simulink model "sedemo_tank_filling_station"  (Simulink 7.5)
settings: Solver=ode45  StartTime=0.0  StopTime=500  MaxStep=inf  RelTol=1e-3
undefined symbols (not defined in the file or in its folder): des_subsystemblock, des_subsysteminport, des_subsystemoutport, des_subsystemsupportblock
libraries: simeventsgenerators1 x3, simeventsattributes2 x2, simeventstranslate1 x2, simeventssignalmanage1 x2, simeventssink1 x1, simeventsinfo x1, simeventsserver1 x1, simeventsqueue1 x1
settings Model: Creator=The MathWorks Inc.  ExtModeAutoUpdateStatusClock=off
settings SolverCC: ZeroCrossControl=EnableAll
settings DataIOCC: SaveOutput=off  SaveTime=off
settings OptimizationCC: InlineInvariantSignals=on  InitFltsAndDblsToZero=on  EfficientMapNaN2IntZero=off
settings DebuggingCC: AlgebraicLoopMsg=error  SaveWithParameterizedLinksMsg=none  SignalResolutionControl=TryResolveAllWithWarning  SolverPrmCheckMsg=none  MultiTaskDSMMsg=warning  MultiTaskCondExecSysMsg=none  SigSpecEnsureSampleTimeMsg=none  InvalidFcnCallConnMsg=warning  BusObjectLabelMismatch=none  StrictBusMsg=None
settings RTWCC: IncludeERTFirstTime=on
settings GRTTargetCC: TargetFcnLib=ansi_tfl_tmw.mat
settings SimEventsCC: propIdentEventSeed=12345678  propDiagAttribOutput=1  propDiagFcnCallOutput=1  propDiagStatOutput=0

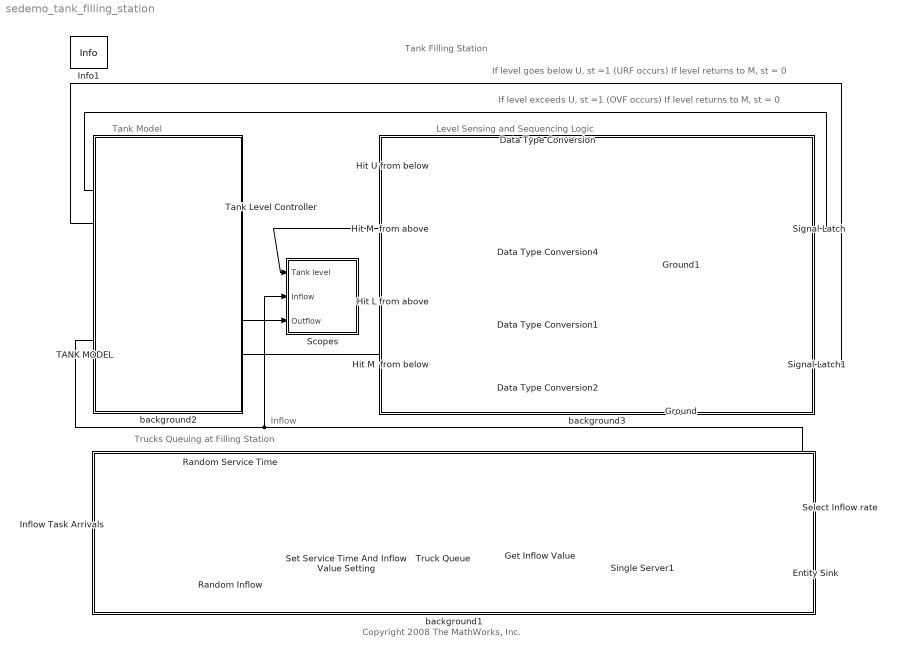
== system sedemo_tank_filling_station ==
  note: If level exceeds U, st =1 (OVF occurs)
      | If level returns to M, st = 0
  note: If level goes below U, st =1 (URF occurs)
      | If level returns to M, st = 0
  note: Tank Filling Station
  note: Trucks Queuing at Filling Station
  note: Tank Model
  note: Level Sensing and Sequencing Logic
  note: Inflow
  note: Copyright 2008 The MathWorks, Inc.
  Data Type Conversion{,1..2,4} (4 alike) : DataTypeConversion  OutDataType=sfix(16)  OutScaling=2^0
  Entity Sink : simeventssink1/Entity Sink  Priority=1  SystemSampleTime=-1  AvailableForArrivals=on  StatNumberArrived=Off
  Get Inflow Value : simeventsattributes2/Get Attribute  Priority=1  DialogController=des_ddg_create  DialogControllerArgs=DataTag2  SystemSampleTime=-1  AttributeName=Inflow  AttributeMissing=Error  AttributeDefaultValue=0  AttributeSendTiming=After entity departure  AttributeTreatAsVector=1  StatNumberDeparted=Off  EvaluatedDefaultAttributeValue={[]}
  Ground : Ground
  Ground1 : Ground
  Hit L from above : HitCross  HitCrossingOffset=1  HitCrossingDirection=falling
  Hit M  from above : HitCross  HitCrossingOffset=3  HitCrossingDirection=falling
  Hit M  from below : HitCross  HitCrossingOffset=3  HitCrossingDirection=rising
  Hit U from below : HitCross  HitCrossingOffset=5  HitCrossingDirection=rising
  Inflow Task Arrivals : simeventsgenerators1/Entity Generators/Time-Based Entity Generator  Priority=1  DialogController=des_ddg_create  DialogControllerArgs=DataTag4  SystemSampleTime=-1  GenerateEntitiesUpon=Intergeneration time from dialog  Distribution=Exponential  Minimum=0  Maximum=8  Mean=1.2  InitialSeed=375501  Period=12  PriorityEntityGeneration=301  GenerateEntityAtSimulationStart=on  ResponseWhenBlocked=Pause generation  ResponseWhenUnblocked=Immediate restart  EntityType=Standard  StatNumberDeparted=Off  StatPendingEntity=Off  StatAverageIntergenerationTime=Off
  Info1 : simeventsinfo/Info  SystemSampleTime=-1
  Random Inflow : simeventsgenerators1/Signal Generators/Event-Based Random Number  SystemSampleTime=-1  distribution=Uniform  meanExp=1  minUnif=10  maxUnif=20  pOneBern=0.25  pSuccessBino=0.5  numTrialBino=1  meanNorm=0  stdNorm=1  minTri=1  maxTri=3  modeTri=2  thresholdLogn=0  scaleLogn=1  shapeLogn=1  pSuccessGeo=0.5  meanPoiss=1  thresholdLogl=0  scaleLogl=1  thresholdGam=0  scaleGam=1  shapeGam=1  minBeta=0  maxBeta=1  shape1Beta=1  shape2Beta=1  minUnid=1  maxUnid=20  numValueUnid=20  thresholdWbl=0  scaleWbl=1  shapeWbl=1  valueVecCont=[0 1]  cdfVecCont=[0 1]  valueVecDisc=[1 2]  probVecDisc=[0.2 0.8]  seed=8023  IsProcessed=on  isConnected=1
  Random Service Time : simeventsgenerators1/Signal Generators/Event-Based Random Number  SystemSampleTime=-1  distribution=Beta  meanExp=1  minUnif=10  maxUnif=20  pOneBern=0.25  pSuccessBino=0.5  numTrialBino=1  meanNorm=0  stdNorm=1  minTri=1  maxTri=3  modeTri=2  thresholdLogn=0  scaleLogn=1  shapeLogn=1  pSuccessGeo=0.5  meanPoiss=1  thresholdLogl=0  scaleLogl=1  thresholdGam=0  scaleGam=1  shapeGam=1  minBeta=.75  maxBeta=1.25  shape1Beta=1  shape2Beta=1  minUnid=1  maxUnid=20  numValueUnid=20  thresholdWbl=0  scaleWbl=1  shapeWbl=1  valueVecCont=[0 1]  cdfVecCont=[0 1]  valueVecDisc=[1 2]  probVecDisc=[0.2 0.8]  seed=9231  IsProcessed=on  isConnected=1
  Scopes : Subsystem
      settings: RequestExecContextInheritance=on
  Select Inflow rate : Subsystem  LoadFcn=des_subsystemblock(gcb, 'load');  InitFcn=des_subsystemblock(gcb, 'init');  StartFcn=des_subsystemblock(gcb, 'start');  StopFcn=des_subsystemblock(gcb, 'stop');
      settings: CopyFcn=des_subsystemblock(gcb, 'copy');  DeleteFcn=des_subsystemblock(gcb, 'delete');  UndoDeleteFcn=des_subsystemblock(gcb, 'undodelete');  ModelCloseFcn=des_subsystemblock(gcb, 'modelclose');  PreSaveFcn=des_subsystemblock(gcb, 'presave');  NameChangeFcn=des_subsystemblock(gcb, 'namechange');  ParentCloseFcn=des_subsystemblock(gcb, 'parentclose');  ErrorFcn=des_subsystemerror
  Set Service Time And Inflow Value Setting : simeventsattributes2/Set Attribute  Priority=1  DialogController=des_ddg_create  DialogControllerArgs=DataTag15  SystemSampleTime=-1  AttributeFrom=Signal port|Signal port  AttributeName=ServiceTime|Inflow  AttributeTreatAsVector=1|1  AttributeValue=1|0  AttributeCreate=on  StatNumberDeparted=Off  EvaluatedAttributeValue={[];[]}
  Signal Latch : simeventssignalmanage1/Signal Latch  Priority=1  SystemSampleTime=-1  InitialMemoryValue=0  WriteMemoryUpon=Change in signal from port wvc  MemoryWriteEdgeOption=Rising  SpecifyWriteEventPriority=on  PriorityMemoryWrite=7100  ReadMemoryUpon=Change in signal from port rvc  MemoryReadEdgeOption=Falling  SpecifyReadEventPriority=on  PriorityMemoryRead=7000  ReportMemoryState=on  ReportMemoryUponWrite=off  ReportMemoryUponRead=off
  Signal Latch1 : simeventssignalmanage1/Signal Latch  Priority=1  SystemSampleTime=-1  InitialMemoryValue=0  WriteMemoryUpon=Change in signal from port wvc  MemoryWriteEdgeOption=Rising  SpecifyWriteEventPriority=on  PriorityMemoryWrite=7100  ReadMemoryUpon=Change in signal from port rvc  MemoryReadEdgeOption=Falling  SpecifyReadEventPriority=on  PriorityMemoryRead=7000  ReportMemoryState=on  ReportMemoryUponWrite=off  ReportMemoryUponRead=off
  Single Server1 : simeventsserver1/Single Server  Priority=1  SystemSampleTime=-1  ServiceTimeFrom=Attribute  ServiceTime=2  AttributeName=ServiceTime  PriorityServiceCompletion=500  PermitPreemption=off  SortingAttributeName=PriorityAttributeName  SortingDirection=Ascending  WriteToAttribute=off  ResidualAttributeName=ResidualServiceTime  CreateAttribute=on  EnableTOPort=off  StatNumberDeparted=Off  StatNumberInBlock=On  StatNumberPreempted=Off  StatPendingEntity=Off  StatAverageWait=Off  StatUtilization=Off  StatNumberTimedout=Off
  TANK MODEL : Subsystem
  Tank Level Controller : Subsystem
  Truck Queue : simeventsqueue1/FIFO Queue  Priority=1  SystemSampleTime=-1  Capacity=2500  EnableTOPort=off  StatNumberDeparted=Off  StatNumberInBlock=Off  StatPendingEntity=Off  StatAverageWait=Off  StatAverageQueueLength=Off  StatNumberTimedout=Off
  background1 : Subsystem
      mask Display: disp('')
  background2 : Subsystem
      mask Display: disp('')
  background3 : Subsystem
      mask Display: disp('')
  wires:
  Signal Latch/1 -> Tank Level Controller/1(OVF state)
  Signal Latch1/1 -> Tank Level Controller/2(URF state)
  Select Inflow rate/1(Inflow) -> TANK MODEL/1(Inflow), Scopes/2(Inflow)
  Hit U from below/1 -> Data Type Conversion/1
  Hit L from above/1 -> Data Type Conversion1/1
  Hit M  from above/1 -> Data Type Conversion4/1
  Tank Level Controller/1(Outflow) -> TANK MODEL/2(Outflow), Scopes/3(Outflow)
  Hit M  from below/1 -> Data Type Conversion2/1
  Ground/1 -> Signal Latch1/3
  Random Inflow/1 -> Set Service Time And Inflow Value Setting/2
  Get Inflow Value/1 -> Select Inflow rate/1(Inflow Value)
  Single Server1/1 -> Select Inflow rate/2(Server State)
  Random Service Time/1 -> Set Service Time And Inflow Value Setting/1
  Data Type Conversion/1 -> Signal Latch/1
  Data Type Conversion4/1 -> Signal Latch/2
  Ground1/1 -> Signal Latch/3
  Data Type Conversion1/1 -> Signal Latch1/1
  Data Type Conversion2/1 -> Signal Latch1/2
  TANK MODEL/1(Tank Level) -> Hit M  from below/1, Hit L from above/1, Hit M  from above/1, Hit U from below/1, Scopes/1(Tank level)
  connections:
  Entity Sink/LConn1 -- Single Server1/RConn1
  Set Service Time And Inflow Value Setting/RConn1 -- Truck Queue/LConn1
  Truck Queue/RConn1 -- Get Inflow Value/LConn1
  Get Inflow Value/RConn1 -- Single Server1/LConn1
  Inflow Task Arrivals/RConn1 -- Set Service Time And Inflow Value Setting/LConn1

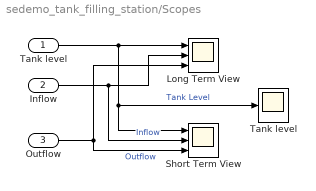
== system sedemo_tank_filling_station/Scopes ==
  Tank level : Inport  OutDataType=sfix(16)  OutScaling=2^0
  Inflow : Inport  Port=2  OutDataType=sfix(16)  OutScaling=2^0
  Outflow : Inport  Port=3  OutDataType=sfix(16)  OutScaling=2^0
  Long Term View : Scope  NumInputPorts=3
      settings: DeleteFcn=simscope BlockIsBeingDestroyed  TickLabels=on  TimeRange=500  YMin=0.5~0~10  YMax=5.5~20~20
  Short Term View : Scope  NumInputPorts=3
      settings: DeleteFcn=simscope BlockIsBeingDestroyed  TickLabels=on  TimeRange=50  YMin=0.5~0~10  YMax=5.5~20~20
  "Tank level " : Scope
      settings: DeleteFcn=simscope BlockIsBeingDestroyed  TickLabels=on  TimeRange=500  YMin=0.5  YMax=5.5  SaveName=ScopeData2
  wires:
  Tank level/1 -> Long Term View/1, Short Term View/1, "Tank level "/1  "Tank Level"
  Inflow/1 -> Long Term View/2, Short Term View/2  "Inflow"
  Outflow/1 -> Short Term View/3, Long Term View/3  "Outflow"

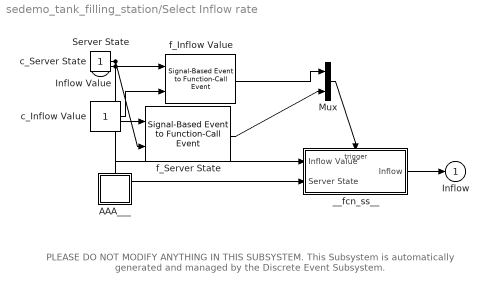
== system sedemo_tank_filling_station/Select Inflow rate ==
  note: PLEASE DO NOT MODIFY ANYTHING IN THIS SUBSYSTEM.
      | This Subsystem is automatically generated and
      | managed by the Discrete Event Subsystem.
  Inflow Value : Inport  DataType=double  OutDataType=sfix(16)  OutScaling=2^0  OutDataTypeStr=double
  Server State : Inport  Port=2  DataType=double  OutDataType=sfix(16)  OutScaling=2^0  OutDataTypeStr=double
  AAA___ : Subsystem  LoadFcn=des_subsystemsupportblock(gcb, 'load');  InitFcn=des_subsystemsupportblock(gcb, 'init');  StartFcn=des_subsystemsupportblock(gcb, 'start');  StopFcn=des_subsystemsupportblock(gcb, 'stop');
      settings: CopyFcn=des_subsystemsupportblock(gcb, 'copy');  DeleteFcn=des_subsystemsupportblock(gcb, 'delete');  UndoDeleteFcn=des_subsystemsupportblock(gcb, 'undodelete');  ModelCloseFcn=des_subsystemsupportblock(gcb, 'modelclose');  PreSaveFcn=des_subsystemsupportblock(gcb, 'presave');  NameChangeFcn=des_subsystemsupportblock(gcb, 'namechange');  OpenFcn=des_subsystemsupportblock(gcb, 'open');  ParentCloseFcn=des_subsystemsupportblock(gcb, 'parentclose');
  Mux : Mux  Inputs=2
  __fcn_ss__ : Subsystem  TreatAsAtomicUnit=on
      settings: PropExecContextOutsideSubsystem=on
  c_Inflow Value : Constant  OutDataType=sfix(16)  OutScaling=2^0
  c_Server State : Constant  OutDataType=sfix(16)  OutScaling=2^0
  f_Inflow Value : simeventstranslate1/Signal-Based Event to Function-Call Event  Priority=1  SystemSampleTime=-1  GenerateFunctionCallUpon=Sample time hit from port ts  SignalEdgeOption=Rising  EnableE1Port=on  EnableF2Port=off  EnableE2Port=off  SpecifyEventPriority=off  PriorityFunctionCall=20  FunctionCallDelayFrom=Dialog  DelayFunctionCall=0  StatNumberF1Calls=Off  StatNumberF2Calls=Off  MaskBlockType=DESS_EVENT_PORT
  f_Server State : simeventstranslate1/Signal-Based Event to Function-Call Event  Priority=1  SystemSampleTime=-1  GenerateFunctionCallUpon=Sample time hit from port ts  SignalEdgeOption=Rising  EnableE1Port=on  EnableF2Port=off  EnableE2Port=off  SpecifyEventPriority=off  PriorityFunctionCall=20  FunctionCallDelayFrom=Dialog  DelayFunctionCall=0  StatNumberF1Calls=Off  StatNumberF2Calls=Off  MaskBlockType=DESS_EVENT_PORT
  Inflow : Outport  OutDataType=sfix(16)  OutScaling=2^0
  wires:
  __fcn_ss__/1(Inflow) -> Inflow/1
  f_Inflow Value/1 -> Mux/1
  c_Inflow Value/1 -> f_Inflow Value/2
  Mux/1 -> __fcn_ss__/Trigger
  f_Server State/1 -> Mux/2
  c_Server State/1 -> f_Server State/2
  Inflow Value/1 -> f_Inflow Value/1, __fcn_ss__/1(Inflow Value)
  Server State/1 -> f_Server State/1, __fcn_ss__/2(Server State)

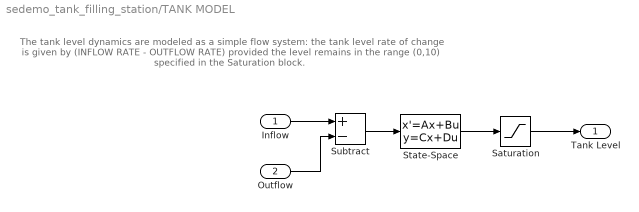
== system sedemo_tank_filling_station/TANK MODEL ==
  note: The tank level dynamics are modeled as a simple flow system:
      |
      |       the tank level rate of change is given by (INFLOW RATE - OUTFLOW RATE)
      |       provided the level remains in the range (0,10) specified in the Saturation block.
  Inflow : Inport  OutDataType=sfix(16)  OutScaling=2^0
  Outflow : Inport  Port=2  OutDataType=sfix(16)  OutScaling=2^0
  Saturation : Saturate  UpperLimit=10  LowerLimit=0
  State-Space : StateSpace  A=0  D=0  X0=2
  Subtract : Sum  Inputs=+-  OutDataType=sfix(16)  OutScaling=2^-10
  Tank Level : Outport  OutDataType=sfix(16)  OutScaling=2^0
  wires:
  Subtract/1 -> State-Space/1
  State-Space/1 -> Saturation/1
  Inflow/1 -> Subtract/1
  Saturation/1 -> Tank Level/1
  Outflow/1 -> Subtract/2

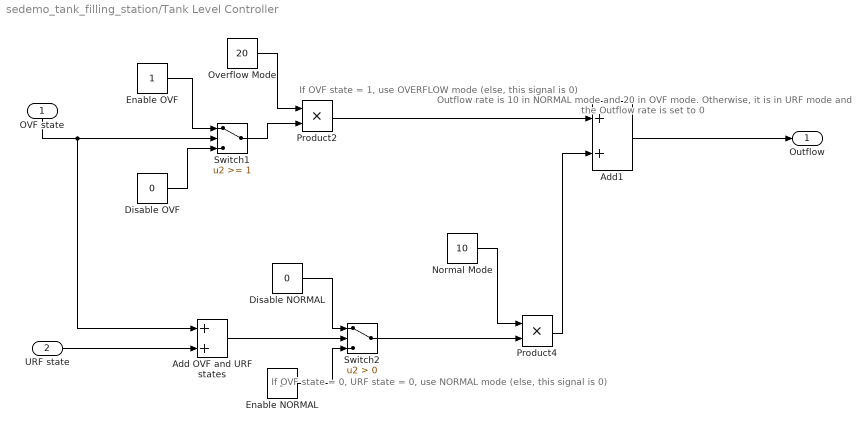
== system sedemo_tank_filling_station/Tank Level Controller ==
  note: If OVF state = 1,
      | use OVERFLOW mode
      | (else, this signal is 0)
  note: If OVF state = 0,
      |   URF state = 0,
      | use NORMAL mode
      | (else, this signal is 0)
  note: Outflow rate is 10 in NORMAL mode
      | and 20 in OVF mode. Otherwise, it is
      | in URF mode and the Outflow rate is set to 0
  OVF state : Inport  OutDataType=sfix(16)  OutScaling=2^0
  URF state : Inport  Port=2  OutDataType=sfix(16)  OutScaling=2^0
  Add OVF and URF states : Sum  OutDataType=sfix(16)  OutScaling=2^-10
  Add1 : Sum  OutDataType=sfix(16)  OutScaling=2^-10
  Disable NORMAL : Constant  Value=0  OutDataType=sfix(16)  OutScaling=2^0
  Disable OVF : Constant  Value=0  OutDataType=sfix(16)  OutScaling=2^0
  Enable NORMAL : Constant  OutDataType=sfix(16)  OutScaling=2^0
  Enable OVF : Constant  OutDataType=sfix(16)  OutScaling=2^0
  Normal Mode : Constant  Value=10  OutDataType=sfix(16)  OutScaling=2^0
  Overflow Mode : Constant  Value=20  OutDataType=sfix(16)  OutScaling=2^0
  Product2 : Product  OutDataType=sfix(16)  OutScaling=2^0  RndMeth=Zero
  Product4 : Product  OutDataType=sfix(16)  OutScaling=2^0  RndMeth=Zero
  Switch1 : Switch  Threshold=1
  Switch2 : Switch  Criteria=u2 > Threshold
  Outflow : Outport  OutDataType=sfix(16)  OutScaling=2^0
  wires:
  Enable OVF/1 -> Switch1/1
  Disable OVF/1 -> Switch1/3
  Switch1/1 -> Product2/2
  Product2/1 -> Add1/1
  Overflow Mode/1 -> Product2/1
  Normal Mode/1 -> Product4/1
  Switch2/1 -> Product4/2
  Product4/1 -> Add1/2
  Add1/1 -> Outflow/1
  Disable NORMAL/1 -> Switch2/1
  Enable NORMAL/1 -> Switch2/3
  Add OVF and URF states/1 -> Switch2/2
  OVF state/1 -> Switch1/2, Add OVF and URF states/1
  URF state/1 -> Add OVF and URF states/2

== system sedemo_tank_filling_station/background1 ==

== system sedemo_tank_filling_station/background2 ==

== system sedemo_tank_filling_station/background3 ==

== system sedemo_tank_filling_station/Select Inflow rate/AAA___ ==

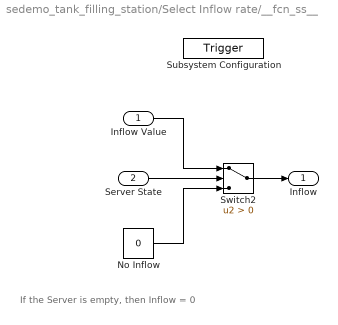
== system sedemo_tank_filling_station/Select Inflow rate/__fcn_ss__ ==
  note: If the Server is empty, then Inflow = 0
  Inflow Value : Inport  LoadFcn=des_subsysteminport(gcb, 'load');  InitFcn=des_subsysteminport(gcb, 'init');  StartFcn=des_subsysteminport(gcb, 'start');  StopFcn=des_subsysteminport(gcb, 'stop');  OutDataType=sfix(16)  OutScaling=2^0  mask(Discrete Event Inport){PermitSubsystemEvents=on, TypeOfEvent=Sample time hit, SignalEdgeOption=Rising, SpecifyEventPriority=off, PrioritySubsystemEvent=20}
      mask prompts: PermitSubsystemEvents "Execute subsystem upon signal-based events"; TypeOfEvent "Type of signal-based event:"; SignalEdgeOption "Type of change in signal value:"; SpecifyEventPriority "Specify event priority for executing subsystem"; PrioritySubsystemEvent "Subsystem execution event priority:"
      mask help: Input port for a Discrete Event Subsystem block. This block can conditionally execute the subsystem upon signal-based events that meet specified criteria.
      mask init:
      | des_subsystemmask(gcb, 'init','apply')
      settings: CopyFcn=des_subsysteminport(gcb, 'copy');  DeleteFcn=des_subsysteminport(gcb, 'delete');  UndoDeleteFcn=des_subsysteminport(gcb, 'undodelete');  ModelCloseFcn=des_subsysteminport(gcb, 'modelclose');  PreSaveFcn=des_subsysteminport(gcb, 'presave');  NameChangeFcn=des_subsysteminport(gcb, 'namechange');  ParentCloseFcn=des_subsysteminport(gcb, 'parentclose');
      mask Help: helpview(simeventsbhelp);
      mask StyleString: checkbox,popup(Change in signal|Trigger|Sample time hit),popup(Rising|Falling|Either),checkbox,edit
      mask CallbackString: des_subsystemmask(gcb, 'cbPermitSubsystemEvents', 'noapply');|des_subsystemmask(gcb,'cbTypeOfEvent','noapply');||des_subsystemmask(gcb, 'cbSpecifyEventPriority', 'noapply');|
  Server State : Inport  LoadFcn=des_subsysteminport(gcb, 'load');  InitFcn=des_subsysteminport(gcb, 'init');  StartFcn=des_subsysteminport(gcb, 'start');  StopFcn=des_subsysteminport(gcb, 'stop');  Port=2  OutDataType=sfix(16)  OutScaling=2^0  mask(Discrete Event Inport){PermitSubsystemEvents=on, TypeOfEvent=Sample time hit, SignalEdgeOption=Rising, SpecifyEventPriority=off, PrioritySubsystemEvent=20}
      mask prompts: PermitSubsystemEvents "Execute subsystem upon signal-based events"; TypeOfEvent "Type of signal-based event:"; SignalEdgeOption "Type of change in signal value:"; SpecifyEventPriority "Specify event priority for executing subsystem"; PrioritySubsystemEvent "Subsystem execution event priority:"
      mask help: Input port for a Discrete Event Subsystem block. This block can conditionally execute the subsystem upon signal-based events that meet specified criteria.
      mask init:
      | des_subsystemmask(gcb, 'init','apply')
      settings: CopyFcn=des_subsysteminport(gcb, 'copy');  DeleteFcn=des_subsysteminport(gcb, 'delete');  UndoDeleteFcn=des_subsysteminport(gcb, 'undodelete');  ModelCloseFcn=des_subsysteminport(gcb, 'modelclose');  PreSaveFcn=des_subsysteminport(gcb, 'presave');  NameChangeFcn=des_subsysteminport(gcb, 'namechange');  ParentCloseFcn=des_subsysteminport(gcb, 'parentclose');
      mask Help: helpview(simeventsbhelp);
      mask StyleString: checkbox,popup(Change in signal|Trigger|Sample time hit),popup(Rising|Falling|Either),checkbox,edit
      mask CallbackString: des_subsystemmask(gcb, 'cbPermitSubsystemEvents', 'noapply');|des_subsystemmask(gcb,'cbTypeOfEvent','noapply');||des_subsystemmask(gcb, 'cbSpecifyEventPriority', 'noapply');|
  Subsystem Configuration : TriggerPort  TriggerType=function-call
      settings: CopyFcn=des_subsystemconfigblock(gcb, 'copy');  DeleteFcn=des_subsystemconfigblock(gcb, 'delete');  UndoDeleteFcn=des_subsystemconfigblock(gcb, 'undodelete');
      mask Type: Subsystem Configuration
      mask Description: Configuration for a Discrete Event Subsystem block. Every discrete event subsystem window must contain exactly one copy of this configuration block. Do not delete this block.
      mask Help: helpview(simeventsbhelp);
      mask Display: disp('Do Not Delete');
  No Inflow : Constant  Value=0  OutDataType=sfix(16)  OutScaling=2^0
  Switch2 : Switch  Criteria=u2 > Threshold
  Inflow : Outport  LoadFcn=des_subsystemoutport(gcb, 'load');  InitFcn=des_subsystemoutport(gcb, 'init');  StartFcn=des_subsystemoutport(gcb, 'start');  StopFcn=des_subsystemoutport(gcb, 'stop');  OutDataType=sfix(16)  OutScaling=2^0
      settings: CopyFcn=des_subsystemoutport(gcb, 'copy');  DeleteFcn=des_subsystemoutport(gcb, 'delete');  UndoDeleteFcn=des_subsystemoutport(gcb, 'undodelete');  ModelCloseFcn=des_subsystemoutport(gcb, 'modelclose');  PreSaveFcn=des_subsystemoutport(gcb, 'presave');  NameChangeFcn=des_subsystemoutport(gcb, 'namechange');  ParentCloseFcn=des_subsystemoutport(gcb, 'parentclose');
      mask Type: Discrete Event Outport
      mask Description: Provide an output port for a Discrete Event Subsystem block.
      mask Help: helpview(simeventsbhelp);
  wires:
  Inflow Value/1 -> Switch2/1
  Server State/1 -> Switch2/2
  No Inflow/1 -> Switch2/3
  Switch2/1 -> Inflow/1
